simulink model "ImpedanceControl"  (R2017a)
settings: Solver=VariableStepAuto  StartTime=0.0  StopTime=10.0  RelTol=1e-3
libraries: mblibv1 x60
(part 2 of 2)

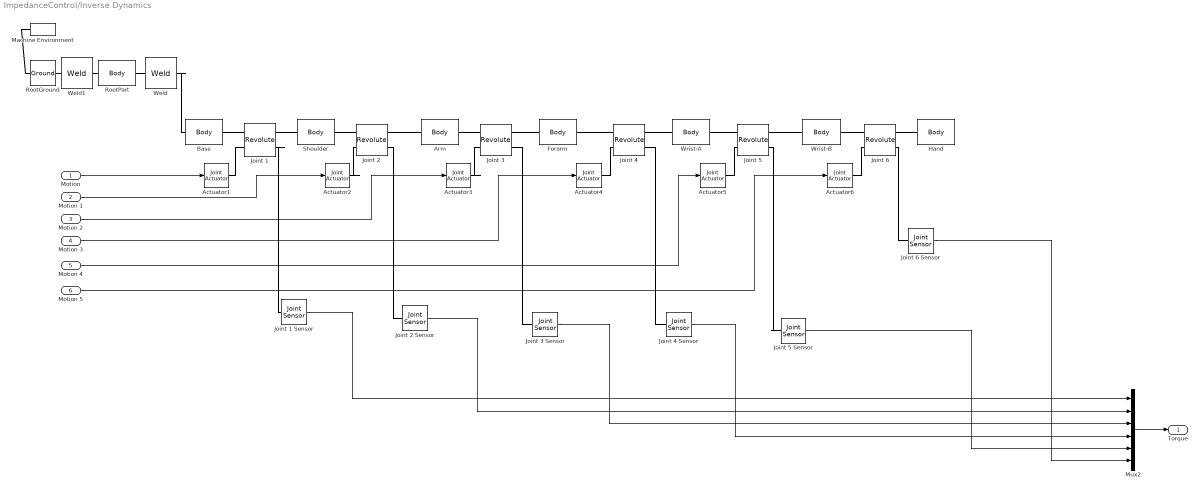
== system ImpedanceControl/Inverse Dynamics  ==
  "Motion " : Inport
  Motion 1 : Inport  Port=2
  Motion 2 : Inport  Port=3
  Motion 3 : Inport  Port=4
  Motion 4 : Inport  Port=5
  Motion 5 : Inport  Port=6
  Actuator{1..6} (6 alike) : mblibv1/Sensors &  Actuators/Joint Actuator  UpdateFromCAD=off  PhysicalDomain=Mechanical  PortType=blob  ActuationStyle=Motion  AngleUnits=deg  ArcVelocityUnits=deg/s  ArcAccelerationUnits=deg/s^2  CoordPositionUnits=m  VelocityUnits=m/s  AccelerationUnits=m/s^2  ForceUnits=N  TorqueUnits=N*m  ActiveIO=on  Width=3  DialogClass=MechanicalActuatorBlock  Primitive=R1  ReferenceFrame=Absolute (World)
      settings: SourceProductName=Simscape Multibody  SourceProductBaseCode=MS
  Arm : mblibv1/Bodies/Body  LConnTagsString=CS2  RConnTagsString=CS3  UpdateFromCAD=on  DialogClass=MechanicalBodyBlock  Mass=1.056  MassUnits=kg  InertiaUnits=kg*m^2  Inertia=[0.0375645,-1.33324e-07,0.000108785;-1.33324e-07,0.0372402,-2.39225e-07;0.000108785,-2.39225e-07,0.00059301]  Shape=Cylinder  ShapeDims=[1 1]  ShapeUnits=m  ShapeUse=false  Density=1  DensityUnits=kg/m^3  DensityUse=false  GraphicsMode=GFXFILE  GraphicsFileName=Jaco_3_7 - arm_ass-1.STL  BodyColorSelMode=COLORPALETTE  BodyColor=[0.752941;0.752941;0.752941]  AttachedToCS=CS1  CG=Right$CG$[0.10282 0.0944444 0.508793]$WORLD$WORLD$m$[0.695251 0.715707 -0.0662524;0.718767 -0.692291 0.0640847;0 -0.092175 -0.995743]$3x3 Transform$rad$WORLD$false$none  WorkingFrames=Right$CS1$[-0.183907 0.105598 0.903425]$WORLD$WORLD$m$[0.695251 0.715707 -0.0662524;0.718767 -0.692291 0.0640847;0 -0.092175 -0.995743]$3x3 Transform$rad$WORLD$false$none#Left$CS2$[0.0767642 0.095252 0.300589]$WORLD$WORLD$m$[1 0 0;0 1 0;0 0 1]$3x3 Transform$rad$WORLD$true$none#Right$CS3$[0.10358 0.0686179 0.708843]$WORLD$WORLD$m$[1 0 0;0 1 0;0 0 1]$3x3 Transform$rad$WORLD$true$none  CGPos=[0.10282 0.0944444 0.508793]  CGRot=[0.695251 0.715707 -0.0662524;0.718767 -0.692291 0.0640847;0 -0.092175 -0.995743]  CS0Pos=[]  CS0Rot=[]  CS1Pos=[-0.183907 0.105598 0.903425]  CS1Rot=[0.695251 0.715707 -0.0662524;0.718767 -0.692291 0.0640847;0 -0.092175 -0.995743]  CS2Pos=[0.0767642 0.095252 0.300589]  CS2Rot=[1 0 0;0 1 0;0 0 1]  CS3Pos=[0.10358 0.0686179 0.708843]  CS3Rot=[1 0 0;0 1 0;0 0 1]  CS4Pos=[]  CS4Rot=[]  CS5Pos=[]  CS5Rot=[]  CS6Pos=[]  CS6Rot=[]  CS7Pos=[]  CS7Rot=[]  CS8Pos=[]  CS8Rot=[]  CS9Pos=[]  CS9Rot=[]  CS10Pos=[]  CS10Rot=[]  CS11Pos=[]  CS11Rot=[]  CS12Pos=[]  CS12Rot=[]  CS13Pos=[]  CS13Rot=[]  CS14Pos=[]  CS14Rot=[]  CS15Pos=[]  CS15Rot=[]  CS16Pos=[]  CS16Rot=[]  CS17Pos=[]  CS17Rot=[]  CS18Pos=[]  CS18Rot=[]  CS19Pos=[]  CS19Rot=[]  CS20Pos=[]  CS20Rot=[]
      settings: SourceProductName=Simscape Multibody  SourceProductBaseCode=MS
  Base : mblibv1/Bodies/Body  LConnTagsString=CS2  RConnTagsString=CS3  UpdateFromCAD=on  DialogClass=MechanicalBodyBlock  Mass=0.570939  MassUnits=kg  InertiaUnits=kg*m^2  Inertia=[0.00175947,1.92772e-07,-3.1782e-05;1.92772e-07,0.00176256,-3.18122e-05;-3.1782e-05,-3.18122e-05,0.000478232]  Shape=Cylinder  ShapeDims=[1 1]  ShapeUnits=m  ShapeUse=false  Density=1  DensityUnits=kg/m^3  DensityUse=false  GraphicsMode=GFXFILE  GraphicsFileName=Jaco_3_7 - base_ass-1.STL  BodyColorSelMode=COLORPALETTE  BodyColor=[0.752941;0.752941;0.752941]  AttachedToCS=CS1  CG=Right$CG$[0.0747134 0.093124 0.128067]$WORLD$WORLD$m$[1 0 0;0 1 0;0 0 1]$3x3 Transform$rad$WORLD$false$none  WorkingFrames=Right$CS1$[0.106448 0.0299726 -0.0762042]$WORLD$WORLD$m$[1 0 0;0 1 0;0 0 1]$3x3 Transform$rad$WORLD$false$none#Left$CS2$[0.0747134 0.093124 0.128067]$WORLD$WORLD$m$[1 0 0;0 1 0;0 0 1]$3x3 Transform$rad$WORLD$true$none#Right$CS3$[0.0753736 0.0938145 0.182089]$WORLD$WORLD$m$[1 0 0;0 1 0;0 0 1]$3x3 Transform$rad$WORLD$true$none  CGPos=[0.0747134 0.093124 0.128067]  CGRot=[1 0 0;0 1 0;0 0 1]  CS0Pos=[]  CS0Rot=[]  CS1Pos=[0.106448 0.0299726 -0.0762042]  CS1Rot=[1 0 0;0 1 0;0 0 1]  CS2Pos=[0.0747134 0.093124 0.128067]  CS2Rot=[1 0 0;0 1 0;0 0 1]  CS3Pos=[0.0753736 0.0938145 0.182089]  CS3Rot=[1 0 0;0 1 0;0 0 1]  CS4Pos=[]  CS4Rot=[]  CS5Pos=[]  CS5Rot=[]  CS6Pos=[]  CS6Rot=[]  CS7Pos=[]  CS7Rot=[]  CS8Pos=[]  CS8Rot=[]  CS9Pos=[]  CS9Rot=[]  CS10Pos=[]  CS10Rot=[]  CS11Pos=[]  CS11Rot=[]  CS12Pos=[]  CS12Rot=[]  CS13Pos=[]  CS13Rot=[]  CS14Pos=[]  CS14Rot=[]  CS15Pos=[]  CS15Rot=[]  CS16Pos=[]  CS16Rot=[]  CS17Pos=[]  CS17Rot=[]  CS18Pos=[]  CS18Rot=[]  CS19Pos=[]  CS19Rot=[]  CS20Pos=[]  CS20Rot=[]
      settings: SourceProductName=Simscape Multibody  SourceProductBaseCode=MS
  Forarm : mblibv1/Bodies/Body  LConnTagsString=CS2  RConnTagsString=CS3  UpdateFromCAD=on  DialogClass=MechanicalBodyBlock  Mass=0.735414  MassUnits=kg  InertiaUnits=kg*m^2  Inertia=[0.00626271,-0.000115651,1.81814e-08;-0.000115651,0.000377159,4.13244e-07;1.81814e-08,4.13244e-07,0.00610747]  Shape=Cylinder  ShapeDims=[1 1]  ShapeUnits=m  ShapeUse=false  Density=1  DensityUnits=kg/m^3  DensityUse=false  GraphicsMode=GFXFILE  GraphicsFileName=Jaco_3_7 - forarm_ass-1.STL  BodyColorSelMode=COLORPALETTE  BodyColor=[0.752941;0.752941;0.752941]  AttachedToCS=CS1  CG=Right$CG$[0.142291 0.0111153 0.740623]$WORLD$WORLD$m$[0.695251 0.650811 0.305076;0.718767 -0.629518 -0.295094;0 0.424443 -0.905455]$3x3 Transform$rad$WORLD$false$none  WorkingFrames=Right$CS1$[-0.0310579 0.0970807 0.899014]$WORLD$WORLD$m$[0.695251 0.650811 0.305076;0.718767 -0.629518 -0.295094;0 0.424443 -0.905455]$3x3 Transform$rad$WORLD$false$none#Left$CS2$[0.10358 0.0686179 0.708843]$WORLD$WORLD$m$[1 0 0;0 1 0;0 0 1]$3x3 Transform$rad$WORLD$true$none#Right$CS3$[0.230802 -0.0700932 0.796915]$WORLD$WORLD$m$[1 0 0;0 1 0;0 0 1]$3x3 Transform$rad$WORLD$true$none  CGPos=[0.142291 0.0111153 0.740623]  CGRot=[0.695251 0.650811 0.305076;0.718767 -0.629518 -0.295094;0 0.424443 -0.905455]  CS0Pos=[]  CS0Rot=[]  CS1Pos=[-0.0310579 0.0970807 0.899014]  CS1Rot=[0.695251 0.650811 0.305076;0.718767 -0.629518 -0.295094;0 0.424443 -0.905455]  CS2Pos=[0.10358 0.0686179 0.708843]  CS2Rot=[1 0 0;0 1 0;0 0 1]  CS3Pos=[0.230802 -0.0700932 0.796915]  CS3Rot=[1 0 0;0 1 0;0 0 1]  CS4Pos=[]  CS4Rot=[]  CS5Pos=[]  CS5Rot=[]  CS6Pos=[]  CS6Rot=[]  CS7Pos=[]  CS7Rot=[]  CS8Pos=[]  CS8Rot=[]  CS9Pos=[]  CS9Rot=[]  CS10Pos=[]  CS10Rot=[]  CS11Pos=[]  CS11Rot=[]  CS12Pos=[]  CS12Rot=[]  CS13Pos=[]  CS13Rot=[]  CS14Pos=[]  CS14Rot=[]  CS15Pos=[]  CS15Rot=[]  CS16Pos=[]  CS16Rot=[]  CS17Pos=[]  CS17Rot=[]  CS18Pos=[]  CS18Rot=[]  CS19Pos=[]  CS19Rot=[]  CS20Pos=[]  CS20Rot=[]
      settings: SourceProductName=Simscape Multibody  SourceProductBaseCode=MS
  Hand : mblibv1/Bodies/Body  LConnTagsString=CS2  UpdateFromCAD=on  DialogClass=MechanicalBodyBlock  Mass=0.395999  MassUnits=kg  InertiaUnits=kg*m^2  Inertia=[0.00124769,-0.000197969,-5.51354e-06;-0.000197969,0.000409818,-2.12169e-05;-5.51354e-06,-2.12169e-05,0.00139509]  Shape=Cylinder  ShapeDims=[1 1]  ShapeUnits=m  ShapeUse=false  Density=1  DensityUnits=kg/m^3  DensityUse=false  GraphicsMode=GFXFILE  GraphicsFileName=Jaco_3_7 - Hand_ass-1.STL  BodyColorSelMode=COLORPALETTE  BodyColor=[0.752941;0.752941;0.752941]  AttachedToCS=CS1  CG=Right$CG$[0.35442 -0.232757 0.799495]$WORLD$WORLD$m$[-0.439555 0.858973 -0.262597;-0.828489 -0.500657 -0.250895;-0.346983 0.107276 0.931716]$3x3 Transform$rad$WORLD$false$none  WorkingFrames=Right$CS1$[0.362295 -0.115327 0.65151]$WORLD$WORLD$m$[-0.439555 0.858973 -0.262597;-0.828489 -0.500657 -0.250895;-0.346983 0.107276 0.931716]$3x3 Transform$rad$WORLD$false$none#Left$CS2$[0.306767 -0.196631 0.795235]$WORLD$WORLD$m$[1 0 0;0 1 0;0 0 1]$3x3 Transform$rad$WORLD$true$none  CGPos=[0.35442 -0.232757 0.799495]  CGRot=[-0.439555 0.858973 -0.262597;-0.828489 -0.500657 -0.250895;-0.346983 0.107276 0.931716]  CS0Pos=[]  CS0Rot=[]  CS1Pos=[0.362295 -0.115327 0.65151]  CS1Rot=[-0.439555 0.858973 -0.262597;-0.828489 -0.500657 -0.250895;-0.346983 0.107276 0.931716]  CS2Pos=[0.306767 -0.196631 0.795235]  CS2Rot=[1 0 0;0 1 0;0 0 1]  CS3Pos=[]  CS3Rot=[]  CS4Pos=[]  CS4Rot=[]  CS5Pos=[]  CS5Rot=[]  CS6Pos=[]  CS6Rot=[]  CS7Pos=[]  CS7Rot=[]  CS8Pos=[]  CS8Rot=[]  CS9Pos=[]  CS9Rot=[]  CS10Pos=[]  CS10Rot=[]  CS11Pos=[]  CS11Rot=[]  CS12Pos=[]  CS12Rot=[]  CS13Pos=[]  CS13Rot=[]  CS14Pos=[]  CS14Rot=[]  CS15Pos=[]  CS15Rot=[]  CS16Pos=[]  CS16Rot=[]  CS17Pos=[]  CS17Rot=[]  CS18Pos=[]  CS18Rot=[]  CS19Pos=[]  CS19Rot=[]  CS20Pos=[]  CS20Rot=[]
      settings: SourceProductName=Simscape Multibody  SourceProductBaseCode=MS
  Joint 1 : mblibv1/Joints/Revolute  LConnTagsString=__newl0|SA1  RConnTagsString=__newr0|SA1  UpdateFromCAD=on  NumSAPorts=2  CutJoint=off  MarkAsCut=off  Primitives=prismatic  PrimitiveProps=R1$World$[0,0,1]$revolute  DialogClass=JointBlock  R1Axis=[0,0,1]
      settings: SourceProductName=Simscape Multibody  SourceProductBaseCode=MS
  Joint 1 Sensor : mblibv1/Sensors &  Actuators/Joint Sensor  UpdateFromCAD=off  PhysicalDomain=Mechanical  PortType=blob  Muxed=off  Pose=off  Angle=off  AngleUnits=deg  ArcVelocity=off  ArcVelocityUnits=deg/s  ArcAcceleration=off  ArcAccelerationUnits=deg/s^2  CoordPosition=on  CoordPositionUnits=m  Velocity=off  VelocityUnits=m/s  Acceleration=off  AccelerationUnits=m/s^2  Quaternion=on  QuaternionDT=off  QuaternionDDT=off  QuaternionUnits=off  OutputVector=[1]  ActiveIO=on  Width=1  DialogClass=MechanicalSensorBlock  Primitive=R1  Force=off  ForceUnits=N  Torque=on  TorqueUnits=N*m  ReferenceFrame=Absolute (World)  ReactionSensedSide=Base  ReactionReferenceFrame=Absolute (World)  ReactionForce=off  ReactionForceUnits=N  ReactionMoment=off  ReactionMomentUnits=N*m
      settings: SourceProductName=Simscape Multibody  SourceProductBaseCode=MS
  Joint 2 : mblibv1/Joints/Revolute  LConnTagsString=__newl0|SA1  RConnTagsString=__newr0|SA1  UpdateFromCAD=on  NumSAPorts=2  CutJoint=off  MarkAsCut=off  Primitives=prismatic  PrimitiveProps=R1$World$[0.695251,0.718767,0]$revolute  DialogClass=JointBlock  R1Axis=[0.695251,0.718767,0]
      settings: SourceProductName=Simscape Multibody  SourceProductBaseCode=MS
  Joint 2 Sensor : mblibv1/Sensors &  Actuators/Joint Sensor  UpdateFromCAD=off  PhysicalDomain=Mechanical  PortType=blob  Muxed=off  Pose=off  Angle=off  AngleUnits=deg  ArcVelocity=off  ArcVelocityUnits=deg/s  ArcAcceleration=off  ArcAccelerationUnits=deg/s^2  CoordPosition=on  CoordPositionUnits=m  Velocity=off  VelocityUnits=m/s  Acceleration=off  AccelerationUnits=m/s^2  Quaternion=on  QuaternionDT=off  QuaternionDDT=off  QuaternionUnits=off  OutputVector=[1]  ActiveIO=on  Width=1  DialogClass=MechanicalSensorBlock  Primitive=R1  Force=off  ForceUnits=N  Torque=on  TorqueUnits=N*m  ReferenceFrame=Absolute (World)  ReactionSensedSide=Base  ReactionReferenceFrame=Absolute (World)  ReactionForce=off  ReactionForceUnits=N  ReactionMoment=off  ReactionMomentUnits=N*m
      settings: SourceProductName=Simscape Multibody  SourceProductBaseCode=MS
  Joint 3 : mblibv1/Joints/Revolute  LConnTagsString=__newl0|SA1  RConnTagsString=__newr0|SA1  UpdateFromCAD=on  NumSAPorts=2  CutJoint=off  MarkAsCut=off  Primitives=prismatic  PrimitiveProps=R1$World$[-0.695251,-0.718767,0]$revolute  DialogClass=JointBlock  R1Axis=[-0.695251,-0.718767,0]
      settings: SourceProductName=Simscape Multibody  SourceProductBaseCode=MS
  Joint 3 Sensor : mblibv1/Sensors &  Actuators/Joint Sensor  UpdateFromCAD=off  PhysicalDomain=Mechanical  PortType=blob  Muxed=off  Pose=off  Angle=off  AngleUnits=deg  ArcVelocity=off  ArcVelocityUnits=deg/s  ArcAcceleration=off  ArcAccelerationUnits=deg/s^2  CoordPosition=on  CoordPositionUnits=m  Velocity=off  VelocityUnits=m/s  Acceleration=off  AccelerationUnits=m/s^2  Quaternion=on  QuaternionDT=off  QuaternionDDT=off  QuaternionUnits=off  OutputVector=[1]  ActiveIO=on  Width=1  DialogClass=MechanicalSensorBlock  Primitive=R1  Force=off  ForceUnits=N  Torque=on  TorqueUnits=N*m  ReferenceFrame=Absolute (World)  ReactionSensedSide=Base  ReactionReferenceFrame=Absolute (World)  ReactionForce=off  ReactionForceUnits=N  ReactionMoment=off  ReactionMomentUnits=N*m
      settings: SourceProductName=Simscape Multibody  SourceProductBaseCode=MS
  Joint 4 : mblibv1/Joints/Revolute  LConnTagsString=__newl0|SA1  RConnTagsString=__newr0|SA1  UpdateFromCAD=on  NumSAPorts=2  CutJoint=off  MarkAsCut=off  Primitives=prismatic  PrimitiveProps=R1$World$[0.650811,-0.629518,0.424443]$revolute  DialogClass=JointBlock  R1Axis=[0.650811,-0.629518,0.424443]
      settings: SourceProductName=Simscape Multibody  SourceProductBaseCode=MS
  Joint 4 Sensor : mblibv1/Sensors &  Actuators/Joint Sensor  UpdateFromCAD=off  PhysicalDomain=Mechanical  PortType=blob  Muxed=off  Pose=off  Angle=off  AngleUnits=deg  ArcVelocity=off  ArcVelocityUnits=deg/s  ArcAcceleration=off  ArcAccelerationUnits=deg/s^2  CoordPosition=on  CoordPositionUnits=m  Velocity=off  VelocityUnits=m/s  Acceleration=off  AccelerationUnits=m/s^2  Quaternion=on  QuaternionDT=off  QuaternionDDT=off  QuaternionUnits=off  OutputVector=[1]  ActiveIO=on  Width=1  DialogClass=MechanicalSensorBlock  Primitive=R1  Force=off  ForceUnits=N  Torque=on  TorqueUnits=N*m  ReferenceFrame=Absolute (World)  ReactionSensedSide=Base  ReactionReferenceFrame=Absolute (World)  ReactionForce=off  ReactionForceUnits=N  ReactionMoment=off  ReactionMomentUnits=N*m
      settings: SourceProductName=Simscape Multibody  SourceProductBaseCode=MS
  Joint 5 : mblibv1/Joints/Revolute  LConnTagsString=__newl0|SA1  RConnTagsString=__newr0|SA1  UpdateFromCAD=on  NumSAPorts=2  CutJoint=off  MarkAsCut=off  Primitives=prismatic  PrimitiveProps=R1$World$[0.15169,-0.946456,-0.284976]$revolute  DialogClass=JointBlock  R1Axis=[0.15169,-0.946456,-0.284976]
      settings: SourceProductName=Simscape Multibody  SourceProductBaseCode=MS
  Joint 5 Sensor : mblibv1/Sensors &  Actuators/Joint Sensor  UpdateFromCAD=off  PhysicalDomain=Mechanical  PortType=blob  Muxed=off  Pose=off  Angle=off  AngleUnits=deg  ArcVelocity=off  ArcVelocityUnits=deg/s  ArcAcceleration=off  ArcAccelerationUnits=deg/s^2  CoordPosition=on  CoordPositionUnits=m  Velocity=off  VelocityUnits=m/s  Acceleration=off  AccelerationUnits=m/s^2  Quaternion=on  QuaternionDT=off  QuaternionDDT=off  QuaternionUnits=off  OutputVector=[1]  ActiveIO=on  Width=1  DialogClass=MechanicalSensorBlock  Primitive=R1  Force=off  ForceUnits=N  Torque=on  TorqueUnits=N*m  ReferenceFrame=Absolute (World)  ReactionSensedSide=Base  ReactionReferenceFrame=Absolute (World)  ReactionForce=off  ReactionForceUnits=N  ReactionMoment=off  ReactionMomentUnits=N*m
      settings: SourceProductName=Simscape Multibody  SourceProductBaseCode=MS
  Joint 6 : mblibv1/Joints/Revolute  LConnTagsString=__newl0|SA1  RConnTagsString=__newr0|SA1  UpdateFromCAD=on  NumSAPorts=2  CutJoint=off  MarkAsCut=off  Primitives=prismatic  PrimitiveProps=R1$World$[0.858973,-0.500657,0.107276]$revolute  DialogClass=JointBlock  R1Axis=[0.858973,-0.500657,0.107276]
      settings: SourceProductName=Simscape Multibody  SourceProductBaseCode=MS
  Joint 6 Sensor : mblibv1/Sensors &  Actuators/Joint Sensor  UpdateFromCAD=off  PhysicalDomain=Mechanical  PortType=blob  Muxed=off  Pose=off  Angle=off  AngleUnits=deg  ArcVelocity=off  ArcVelocityUnits=deg/s  ArcAcceleration=off  ArcAccelerationUnits=deg/s^2  CoordPosition=on  CoordPositionUnits=m  Velocity=off  VelocityUnits=m/s  Acceleration=off  AccelerationUnits=m/s^2  Quaternion=on  QuaternionDT=off  QuaternionDDT=off  QuaternionUnits=off  OutputVector=[1]  ActiveIO=on  Width=1  DialogClass=MechanicalSensorBlock  Primitive=R1  Force=off  ForceUnits=N  Torque=on  TorqueUnits=N*m  ReferenceFrame=Absolute (World)  ReactionSensedSide=Base  ReactionReferenceFrame=Absolute (World)  ReactionForce=off  ReactionForceUnits=N  ReactionMoment=off  ReactionMomentUnits=N*m
      settings: SourceProductName=Simscape Multibody  SourceProductBaseCode=MS
  Machine Environment : mblibv1/Bodies/Machine Environment  PortType=env  PhysicalDomain=Mechanical  DialogTemplateClass=MECH.MachineEnvironment  SyncWhenCopied=off  Gravity=[0 0 -9.81]  GravityUnits=m/s^2  GravityAsSignal=off  Dimensionality=Auto-detect  AnalysisType=Inverse dynamics  LinearAssemblyTolerance=1e-3  LinearAssemblyToleranceUnits=m  AngularAssemblyTolerance=1e-3  AngularAssemblyToleranceUnits=rad  ConstraintSolverType=Stabilizing  ConstraintRelTolerance=1e-4  ConstraintAbsTolerance=1e-4  UseRobustSingularityHandling=off  RedundancyAnalysisToleranceType=Automatically select tolerance  RedundancyAnalysisTolerance=1e-14  StatePerturbationType=Fixed  PerturbationSize=1e-5  VisualizeMachine=on  BodyVisualizationType=Use model default body geometries  BodyColorSelMode=Use model default  DefaultBodyColor=[1 0 0]
      settings: SourceProductName=Simscape Multibody  SourceProductBaseCode=MS
  Mux2 : Mux  Inputs=6
  RootGround : mblibv1/Bodies/Ground  UpdateFromCAD=on  LeftPortType=env  RightPortType=workingframe  PhysicalDomain=Mechanical  DialogClass=GroundBlock  CoordPosition=[0.154743,0.00421299,0.535333]  CoordPositionUnits=m  StateVectorMgrId=-1  MachineId=[0 0]  ShowEnvPort=on  ParameterChecksum=[2113353881, 666478824, 1095862328, 2132002380]  TopologyChecksum=[2383253151, 3882554260, 534595173, 222725373]
      settings: SourceProductName=Simscape Multibody  SourceProductBaseCode=MS
  RootPart : mblibv1/Bodies/Body  LConnTagsString=CS3  RConnTagsString=CS2  UpdateFromCAD=on  DialogClass=MechanicalBodyBlock  Mass=0  MassUnits=kg  InertiaUnits=kg*m^2  Inertia=[0,0,0;0,0,0;0,0,0]  Shape=Cylinder  ShapeDims=[1 1]  ShapeUnits=m  ShapeUse=false  Density=1  DensityUnits=kg/m^3  DensityUse=false  GraphicsMode=MACHINE_DEFAULT  BodyColorSelMode=MACHINE_DEFAULT  BodyColor=[1;0;0]  AttachedToCS=CS1  CG=Right$CG$[0.154743 0.00421299 0.535333]$WORLD$WORLD$m$[1 0 0;0 1 0;0 0 1]$3x3 Transform$rad$WORLD$false$none  WorkingFrames=Right$CS1$[0 0 0]$WORLD$WORLD$m$[1 0 0;0 1 0;0 0 1]$3x3 Transform$rad$WORLD$false$none#Right$CS2$[0.0747134 0.093124 0.128067]$WORLD$WORLD$m$[1 0 0;0 1 0;0 0 1]$3x3 Transform$rad$WORLD$true$none#Left$CS3$[0.154743 0.00421299 0.535333]$WORLD$WORLD$m$[1 0 0;0 1 0;0 0 1]$3x3 Transform$rad$WORLD$true$none  CGPos=[0.154743 0.00421299 0.535333]  CGRot=[1 0 0;0 1 0;0 0 1]  CS0Pos=[]  CS0Rot=[]  CS1Pos=[0 0 0]  CS1Rot=[1 0 0;0 1 0;0 0 1]  CS2Pos=[0.0747134 0.093124 0.128067]  CS2Rot=[1 0 0;0 1 0;0 0 1]  CS3Pos=[0.154743 0.00421299 0.535333]  CS3Rot=[1 0 0;0 1 0;0 0 1]  CS4Pos=[]  CS4Rot=[]  CS5Pos=[]  CS5Rot=[]  CS6Pos=[]  CS6Rot=[]  CS7Pos=[]  CS7Rot=[]  CS8Pos=[]  CS8Rot=[]  CS9Pos=[]  CS9Rot=[]  CS10Pos=[]  CS10Rot=[]  CS11Pos=[]  CS11Rot=[]  CS12Pos=[]  CS12Rot=[]  CS13Pos=[]  CS13Rot=[]  CS14Pos=[]  CS14Rot=[]  CS15Pos=[]  CS15Rot=[]  CS16Pos=[]  CS16Rot=[]  CS17Pos=[]  CS17Rot=[]  CS18Pos=[]  CS18Rot=[]  CS19Pos=[]  CS19Rot=[]  CS20Pos=[]  CS20Rot=[]
      settings: SourceProductName=Simscape Multibody  SourceProductBaseCode=MS
  Shoulder : mblibv1/Bodies/Body  LConnTagsString=CS3  RConnTagsString=CS2  UpdateFromCAD=on  DialogClass=MechanicalBodyBlock  Mass=0.813994  MassUnits=kg  InertiaUnits=kg*m^2  Inertia=[0.0026546,0.000304923,5.38935e-08;0.000304923,0.000595598,-3.17242e-07;5.38935e-08,-3.17242e-07,0.00258406]  Shape=Cylinder  ShapeDims=[1 1]  ShapeUnits=m  ShapeUse=false  Density=1  DensityUnits=kg/m^3  DensityUse=false  GraphicsMode=GFXFILE  GraphicsFileName=Jaco_3_7 - shoulder_ass-1.STL  BodyColorSelMode=COLORPALETTE  BodyColor=[0.752941;0.752941;0.752941]  AttachedToCS=CS1  CG=Right$CG$[0.0698164 0.0880634 0.250193]$WORLD$WORLD$m$[0.695251 0 0.718767;0.718767 0 -0.695251;0 1 0]$3x3 Transform$rad$WORLD$false$none  WorkingFrames=Right$CS1$[-0.0564522 0.142463 0.184725]$WORLD$WORLD$m$[0.695251 0 0.718767;0.718767 0 -0.695251;0 1 0]$3x3 Transform$rad$WORLD$false$none#Right$CS2$[0.0767642 0.095252 0.300589]$WORLD$WORLD$m$[1 0 0;0 1 0;0 0 1]$3x3 Transform$rad$WORLD$true$none#Left$CS3$[0.0753736 0.0938145 0.182089]$WORLD$WORLD$m$[1 0 0;0 1 0;0 0 1]$3x3 Transform$rad$WORLD$true$none  CGPos=[0.0698164 0.0880634 0.250193]  CGRot=[0.695251 0 0.718767;0.718767 0 -0.695251;0 1 0]  CS0Pos=[]  CS0Rot=[]  CS1Pos=[-0.0564522 0.142463 0.184725]  CS1Rot=[0.695251 0 0.718767;0.718767 0 -0.695251;0 1 0]  CS2Pos=[0.0767642 0.095252 0.300589]  CS2Rot=[1 0 0;0 1 0;0 0 1]  CS3Pos=[0.0753736 0.0938145 0.182089]  CS3Rot=[1 0 0;0 1 0;0 0 1]  CS4Pos=[]  CS4Rot=[]  CS5Pos=[]  CS5Rot=[]  CS6Pos=[]  CS6Rot=[]  CS7Pos=[]  CS7Rot=[]  CS8Pos=[]  CS8Rot=[]  CS9Pos=[]  CS9Rot=[]  CS10Pos=[]  CS10Rot=[]  CS11Pos=[]  CS11Rot=[]  CS12Pos=[]  CS12Rot=[]  CS13Pos=[]  CS13Rot=[]  CS14Pos=[]  CS14Rot=[]  CS15Pos=[]  CS15Rot=[]  CS16Pos=[]  CS16Rot=[]  CS17Pos=[]  CS17Rot=[]  CS18Pos=[]  CS18Rot=[]  CS19Pos=[]  CS19Rot=[]  CS20Pos=[]  CS20Rot=[]
      settings: SourceProductName=Simscape Multibody  SourceProductBaseCode=MS
  Weld : mblibv1/Joints/Weld  LConnTagsString=__newl0  RConnTagsString=__newr0  UpdateFromCAD=on  NumSAPorts=0  CutJoint=off  MarkAsCut=off  Primitives=weld  PrimitiveProps=W$WORLD$[0.57735,0.57735,0.57735]$weld  DialogClass=JointBlock  WAxis=[0.57735,0.57735,0.57735]
      settings: SourceProductName=Simscape Multibody  SourceProductBaseCode=MS
  Weld1 : mblibv1/Joints/Weld  LConnTagsString=__newl0  RConnTagsString=__newr0  UpdateFromCAD=on  NumSAPorts=0  CutJoint=off  MarkAsCut=off  Primitives=weld  PrimitiveProps=W$WORLD$[0.57735,0.57735,0.57735]$weld  DialogClass=JointBlock  WAxis=[0.57735,0.57735,0.57735]
      settings: SourceProductName=Simscape Multibody  SourceProductBaseCode=MS
  Wrist-A : mblibv1/Bodies/Body  LConnTagsString=CS3  RConnTagsString=CS2  UpdateFromCAD=on  DialogClass=MechanicalBodyBlock  Mass=0.44698  MassUnits=kg  InertiaUnits=kg*m^2  Inertia=[0.000407036,-3.06246e-08,5.0605e-09;-3.06246e-08,0.000239744,-8.7175e-05;5.0605e-09,-8.7175e-05,0.000376656]  Shape=Cylinder  ShapeDims=[1 1]  ShapeUnits=m  ShapeUse=false  Density=1  DensityUnits=kg/m^3  DensityUse=false  GraphicsMode=GFXFILE  GraphicsFileName=Jaco_3_7 - wrist1_ass-1.STL  BodyColorSelMode=COLORPALETTE  BodyColor=[0.752941;0.752941;0.752941]  AttachedToCS=CS1  CG=Right$CG$[0.251866 -0.101707 0.805258]$WORLD$WORLD$m$[0.709409 0.650811 -0.270524;0.30501 -0.629518 -0.714616;-0.63538 0.424443 -0.64509]$3x3 Transform$rad$WORLD$false$none  WorkingFrames=Right$CS1$[0.228148 -0.0304193 0.852839]$WORLD$WORLD$m$[0.709409 0.650811 -0.270524;0.30501 -0.629518 -0.714616;-0.63538 0.424443 -0.64509]$3x3 Transform$rad$WORLD$false$none#Right$CS2$[0.264276 -0.136155 0.802577]$WORLD$WORLD$m$[1 0 0;0 1 0;0 0 1]$3x3 Transform$rad$WORLD$true$none#Left$CS3$[0.230802 -0.0700932 0.796915]$WORLD$WORLD$m$[1 0 0;0 1 0;0 0 1]$3x3 Transform$rad$WORLD$true$none  CGPos=[0.251866 -0.101707 0.805258]  CGRot=[0.709409 0.650811 -0.270524;0.30501 -0.629518 -0.714616;-0.63538 0.424443 -0.64509]  CS0Pos=[]  CS0Rot=[]  CS1Pos=[0.228148 -0.0304193 0.852839]  CS1Rot=[0.709409 0.650811 -0.270524;0.30501 -0.629518 -0.714616;-0.63538 0.424443 -0.64509]  CS2Pos=[0.264276 -0.136155 0.802577]  CS2Rot=[1 0 0;0 1 0;0 0 1]  CS3Pos=[0.230802 -0.0700932 0.796915]  CS3Rot=[1 0 0;0 1 0;0 0 1]  CS4Pos=[]  CS4Rot=[]  CS5Pos=[]  CS5Rot=[]  CS6Pos=[]  CS6Rot=[]  CS7Pos=[]  CS7Rot=[]  CS8Pos=[]  CS8Rot=[]  CS9Pos=[]  CS9Rot=[]  CS10Pos=[]  CS10Rot=[]  CS11Pos=[]  CS11Rot=[]  CS12Pos=[]  CS12Rot=[]  CS13Pos=[]  CS13Rot=[]  CS14Pos=[]  CS14Rot=[]  CS15Pos=[]  CS15Rot=[]  CS16Pos=[]  CS16Rot=[]  CS17Pos=[]  CS17Rot=[]  CS18Pos=[]  CS18Rot=[]  CS19Pos=[]  CS19Rot=[]  CS20Pos=[]  CS20Rot=[]
      settings: SourceProductName=Simscape Multibody  SourceProductBaseCode=MS
  Wrist-B : mblibv1/Bodies/Body  LConnTagsString=CS3  RConnTagsString=CS2  UpdateFromCAD=on  DialogClass=MechanicalBodyBlock  Mass=0.44698  MassUnits=kg  InertiaUnits=kg*m^2  Inertia=[0.000407036,-3.06246e-08,5.0605e-09;-3.06246e-08,0.000239744,-8.7175e-05;5.0605e-09,-8.7175e-05,0.000376656]  Shape=Cylinder  ShapeDims=[1 1]  ShapeUnits=m  ShapeUse=false  Density=1  DensityUnits=kg/m^3  DensityUse=false  GraphicsMode=GFXFILE  GraphicsFileName=Jaco_3_7 - wrist2_ass-1.STL  BodyColorSelMode=COLORPALETTE  BodyColor=[0.752941;0.752941;0.752941]  AttachedToCS=CS1  CG=Right$CG$[0.28076 -0.170724 0.795794]$WORLD$WORLD$m$[-0.298122 0.15169 0.942398;-0.318695 -0.946456 0.0515257;0.899754 -0.284976 0.330502]$3x3 Transform$rad$WORLD$false$none  WorkingFrames=Right$CS1$[0.211333 -0.128563 0.759589]$WORLD$WORLD$m$[-0.298122 0.15169 0.942398;-0.318695 -0.946456 0.0515257;0.899754 -0.284976 0.330502]$3x3 Transform$rad$WORLD$false$none#Right$CS2$[0.306767 -0.196631 0.795235]$WORLD$WORLD$m$[1 0 0;0 1 0;0 0 1]$3x3 Transform$rad$WORLD$true$none#Left$CS3$[0.264276 -0.136155 0.802577]$WORLD$WORLD$m$[1 0 0;0 1 0;0 0 1]$3x3 Transform$rad$WORLD$true$none  CGPos=[0.28076 -0.170724 0.795794]  CGRot=[-0.298122 0.15169 0.942398;-0.318695 -0.946456 0.0515257;0.899754 -0.284976 0.330502]  CS0Pos=[]  CS0Rot=[]  CS1Pos=[0.211333 -0.128563 0.759589]  CS1Rot=[-0.298122 0.15169 0.942398;-0.318695 -0.946456 0.0515257;0.899754 -0.284976 0.330502]  CS2Pos=[0.306767 -0.196631 0.795235]  CS2Rot=[1 0 0;0 1 0;0 0 1]  CS3Pos=[0.264276 -0.136155 0.802577]  CS3Rot=[1 0 0;0 1 0;0 0 1]  CS4Pos=[]  CS4Rot=[]  CS5Pos=[]  CS5Rot=[]  CS6Pos=[]  CS6Rot=[]  CS7Pos=[]  CS7Rot=[]  CS8Pos=[]  CS8Rot=[]  CS9Pos=[]  CS9Rot=[]  CS10Pos=[]  CS10Rot=[]  CS11Pos=[]  CS11Rot=[]  CS12Pos=[]  CS12Rot=[]  CS13Pos=[]  CS13Rot=[]  CS14Pos=[]  CS14Rot=[]  CS15Pos=[]  CS15Rot=[]  CS16Pos=[]  CS16Rot=[]  CS17Pos=[]  CS17Rot=[]  CS18Pos=[]  CS18Rot=[]  CS19Pos=[]  CS19Rot=[]  CS20Pos=[]  CS20Rot=[]
      settings: SourceProductName=Simscape Multibody  SourceProductBaseCode=MS
  "Torque " : Outport
  wires:
  Motion 1/1 -> Actuator2/1
  Motion 2/1 -> Actuator3/1
  Motion 3/1 -> Actuator4/1
  Motion 4/1 -> Actuator5/1
  Motion 5/1 -> Actuator6/1
  Joint 3 Sensor/1 -> Mux2/3
  Joint 6 Sensor/1 -> Mux2/6
  "Motion "/1 -> Actuator1/1
  Mux2/1 -> "Torque "/1
  Joint 1 Sensor/1 -> Mux2/1
  Joint 2 Sensor/1 -> Mux2/2
  Joint 4 Sensor/1 -> Mux2/4
  Joint 5 Sensor/1 -> Mux2/5
  connections:
  Actuator5/RConn1 -- Joint 5/LConn2
  Shoulder/RConn1 -- Joint 2/LConn1
  Joint 3 Sensor/LConn1 -- Joint 3/RConn2
  Weld/RConn1 -- Base/LConn1
  Joint 3/RConn1 -- Forarm/LConn1
  Joint 5/RConn1 -- Wrist-B/LConn1
  Joint 6/RConn1 -- Hand/LConn1
  Joint 6 Sensor/LConn1 -- Joint 6/RConn2
  Joint 2/RConn1 -- Arm/LConn1
  Actuator3/RConn1 -- Joint 3/LConn2
  Joint 5 Sensor/LConn1 -- Joint 5/RConn2
  Joint 4 Sensor/LConn1 -- Joint 4/RConn2
  Arm/RConn1 -- Joint 3/LConn1
  Actuator6/RConn1 -- Joint 6/LConn2
  Actuator4/RConn1 -- Joint 4/LConn2
  Joint 1/RConn1 -- Shoulder/LConn1
  RootPart/RConn1 -- Weld/LConn1
  Base/RConn1 -- Joint 1/LConn1
  Wrist-A/RConn1 -- Joint 5/LConn1
  Wrist-B/RConn1 -- Joint 6/LConn1
  Weld1/RConn1 -- RootPart/LConn1
  Joint 4/RConn1 -- Wrist-A/LConn1
  Forarm/RConn1 -- Joint 4/LConn1
  Joint 2 Sensor/LConn1 -- Joint 2/RConn2
  RootGround/RConn1 -- Weld1/LConn1
  Actuator2/RConn1 -- Joint 2/LConn2
  Joint 1/LConn2 -- Actuator1/RConn1
  Joint 1/RConn2 -- Joint 1 Sensor/LConn1
  Machine Environment/RConn1 -- RootGround/LConn1

== matlab function ImpedanceControl/MATLAB Function1 ==
  data: q input; We output; dq input
function We  = Jacobian_angular_velocities(q,dq)
%JACOBIANW
%    B = JACOBIANW(Q1,Q2,Q3,Q4,Q5)

%    This function was generated by the Symbolic Math Toolbox version 7.2.
%    23-Apr-2017 14:55:34

q=num2cell(q);
[q1,q2,q3,q4,q5,~]=deal(q{:});
%dq=num2cell(dq);
%[dq1,dq2,dq3,dq4,dq5,dq6]=deal(dq{:});

t2 = sin(q1);
t3 = cos(q1);
t4 = cos(q2);
t5 = sin(q3);
t6 = t3.*t4.*t5;
t7 = cos(q3);
t8 = sin(q2);
t13 = t3.*t7.*t8;
t9 = t6-t13;
t10 = pi.*(1.1e1./3.6e1);
t11 = sin(t10);
t12 = cos(t10);
t14 = t9.*t12;
t15 = cos(q4);
t16 = t2.*t11.*t15;
t17 = sin(q4);
t18 = t3.*t4.*t7;
t19 = t3.*t5.*t8;
t20 = t18+t19;
t21 = t11.*t17.*t20;
t22 = t14+t16+t21;
t23 = q2-q3;
t24 = sin(q5);
t25 = t2.*t17;
t26 = cos(q5);
t27 = t2.*t12.*t15;
t28 = sin(t23);
t29 = cos(t23);
t30 = t2.*t4.*t5;
t32 = t2.*t7.*t8;
t31 = t30-t32;
t33 = t12.*t31;
t34 = t2.*t5.*t8;
t35 = t2.*t4.*t7;
t36 = t34+t35;
t37 = t11.*t17.*t36;
t39 = t3.*t11.*t15;
t38 = t33+t37-t39;
t40 = t3.*t17;
t41 = t3.*t12.*t15;
t42 = t4.*t7;
t43 = t5.*t8;
t44 = t42+t43;
t45 = t12.*t44;
t46 = t4.*t5;
t49 = t7.*t8;
t47 = t46-t49;
t48 = t45-t11.*t17.*t47;
B = reshape([t2,-t3,0.0,-t2,t3,0.0,t9,t31,t44,t22,t38,t48,t12.*t22+t11.*t26.*(t27-t9.*t11+t12.*t17.*t20)-t11.*t24.*(t25-t15.*t20),t12.*t38-t11.*t26.*(t41+t11.*t31-t12.*t17.*t36)+t11.*t24.*(t40+t15.*t36),t12.*t48-t11.*t26.*(t11.*t44+t12.*t17.*t47)-t11.*t15.*t24.*t47,-t12.*(t16-t3.*t12.*t28+t3.*t11.*t17.*t29)-t11.*t26.*(t27+t3.*t11.*t28+t3.*t12.*t17.*t29)-t11.*t24.*(-t25+t3.*t4.*t7.*t15+t3.*t5.*t8.*t15),t12.*(t39+t2.*t12.*t28-t2.*t11.*t17.*t29)-t11.*t26.*(-t41+t2.*t11.*t28+t2.*t12.*t17.*t29)-t11.*t24.*(t40+t2.*t4.*t7.*t15+t2.*t5.*t8.*t15),-t12.*(t12.*t29+t11.*t17.*t28)+t11.*t26.*(t11.*t29-t12.*t17.*t28)-t11.*t15.*t24.*t28],[3,6]);
We=B*dq;

== matlab function ImpedanceControl/MATLAB Function ==
  data: q input; Oe output; Re output
function [ Oe, Re ] = DirectKinematics(q)
% DirectKinematics
%    [ Oe, Re ] = DirectKinematics(q)
%    This function was generated by the Symbolic Math Toolbox version 7.2.
%    23-Apr-2017 13:45:31

q=num2cell(q);
[q1,q2,q3,q4,q5,q6]=deal(q{:});

t2 = q1+q2;
t3 = cos(t2);
t4 = q3+q4;
t5 = sin(t2);
t6 = cos(q5);
t7 = cos(t4);
t8 = sin(q5);
t9 = sin(q6);
t10 = cos(q6);
t11 = sin(t4);
t12 = t3.*t11.*4.698463103929542e-1;
t13 = t3.*t7.*t8.*4.698463103929542e-1;
t14 = t5.*t11.*4.698463103929542e-1;
t15 = t3.*t8;
t16 = t15-t5.*t6.*t7;
t17 = t3.*t6.*4.698463103929542e-1;
t18 = t5.*t7.*t8.*4.698463103929542e-1;
t19 = cos(q3);
T06 = reshape([t10.*(t5.*t8+t3.*t6.*t7)-t9.*(t5.*t6.*(-5.735764363510462e-1)+t3.*t11.*8.191520442889917e-1+t3.*t7.*t8.*5.735764363510462e-1),-t10.*t16-t9.*(t3.*t6.*5.735764363510462e-1+t5.*t11.*8.191520442889917e-1+t5.*t7.*t8.*5.735764363510462e-1),t7.*t9.*(-8.191520442889917e-1)-t6.*t10.*t11+t8.*t9.*t11.*5.735764363510462e-1,0.0,-t12-t10.*(t12-t5.*t6.*3.289899283371657e-1+t3.*t7.*t8.*3.289899283371657e-1)-t9.*(t5.*t8.*5.735764363510462e-1+t3.*t6.*t7.*5.735764363510462e-1)-t5.*t6.*6.710100716628342e-1+t3.*t7.*t8.*6.710100716628342e-1,-t14-t10.*(t14+t3.*t6.*3.289899283371657e-1+t5.*t7.*t8.*3.289899283371657e-1)+t9.*(t3.*t8.*5.735764363510462e-1-t5.*t6.*t7.*5.735764363510462e-1)+t3.*t6.*6.710100716628342e-1+t5.*t7.*t8.*6.710100716628342e-1,t7.*(-4.698463103929542e-1)-t7.*t10.*4.698463103929542e-1-t8.*t11.*6.710100716628342e-1+t6.*t9.*t11.*5.735764363510462e-1+t8.*t10.*t11.*3.289899283371657e-1,0.0,t13+t10.*(t13-t5.*t6.*4.698463103929542e-1+t3.*t11.*6.710100716628342e-1)-t5.*t6.*4.698463103929542e-1-t3.*t11.*3.289899283371657e-1+t9.*(t5.*t8.*8.191520442889917e-1+t3.*t6.*t7.*8.191520442889917e-1),t17+t18-t5.*t11.*3.289899283371657e-1-t9.*t16.*8.191520442889917e-1+t10.*(t17+t18+t5.*t11.*6.710100716628342e-1),t7.*(-3.289899283371657e-1)+t7.*t10.*6.710100716628342e-1-t8.*t11.*4.698463103929542e-1-t6.*t9.*t11.*8.191520442889917e-1-t8.*t10.*t11.*4.698463103929542e-1,0.0,t5.*(-2.589822393260846e-1)-t5.*t6.*1.724988718349159e-1-t3.*t11.*2.04549489043648e-1+t3.*t19.*(4.1e1./1.0e2)+t3.*t7.*t8.*1.724988718349159e-1,t3.*2.589822393260846e-1+t3.*t6.*1.724988718349159e-1-t5.*t11.*2.04549489043648e-1+t5.*t19.*(4.1e1./1.0e2)+t5.*t7.*t8.*1.724988718349159e-1,t7.*(-2.04549489043648e-1)-sin(q3).*(4.1e1./1.0e2)-t8.*t11.*1.724988718349159e-1+2.755e-1,1.0],[4,4]);
Re=T06(1:3,1:3);
Oe=T06(1:3,4);

== matlab function ImpedanceControl/MATLAB Function2 ==
  data: q input; dOe output; dq input
function dOe = PositionDerivative(q,dq)
%POSITIONDERIVATIVE
%    DOE = POSITIONDERIVATIVE(DQ1,DQ2,DQ3,DQ4,DQ5,Q1,Q2,Q3,Q4,Q5)

%    This function was generated by the Symbolic Math Toolbox version 7.2.
%    23-Apr-2017 15:43:12

q=num2cell(q);
dq=num2cell(dq);
[q1,q2,q3,q4,q5,q6]=deal(q{:});
[dq1,dq2,dq3,dq4,dq5,dq6]=deal(dq{:});

t2 = q1+q2;
t3 = dq1+dq2;
t4 = cos(t2);
t5 = pi.*(1.1e1./7.2e1);
t6 = cos(t5);
t7 = sin(t2);
t8 = pi.*(1.1e1./3.6e1);
t9 = sin(t8);
t10 = cos(t8);
t11 = q3+q4;
t12 = cos(t11);
t13 = cos(q5);
t14 = sin(q5);
t15 = sin(t11);
t16 = dq3+dq4;
t17 = 1.0./t6;
t18 = cos(q3);
t19 = sin(q3);
t20 = t6.*3.374e3;
t21 = t20+7.43e2;
t22 = t6.*4.146e3;
t23 = t22+7.43e2;
t24 = sin(t5);
dOe = [t3.*t4.*(-9.8e-3)-t17.*t21.*(-dq5.*t7.*t9.*t14+t3.*t4.*t9.*t13-t3.*t7.*t10.*t15+t4.*t10.*t12.*t16-dq5.*t4.*t9.*t12.*t13+t3.*t7.*t9.*t12.*t14+t4.*t9.*t14.*t15.*t16).*5.0e-5-dq3.*t4.*t19.*(4.1e1./1.0e2)-t3.*t7.*t18.*(4.1e1./1.0e2)+t3.*t7.*t15.*t17.*7.43e-2-t3.*t4.*t17.*t23.*5.0e-5-t4.*t12.*t16.*t17.*7.43e-2;t3.*t7.*(-9.8e-3)-t17.*t21.*(dq5.*t4.*t9.*t14+t3.*t4.*t10.*t15+t3.*t7.*t9.*t13+t7.*t10.*t12.*t16-dq5.*t7.*t9.*t12.*t13-t3.*t4.*t9.*t12.*t14+t7.*t9.*t14.*t15.*t16).*5.0e-5-dq3.*t7.*t19.*(4.1e1./1.0e2)+t3.*t4.*t18.*(4.1e1./1.0e2)-t3.*t4.*t15.*t17.*7.43e-2-t3.*t7.*t17.*t23.*5.0e-5-t7.*t12.*t16.*t17.*7.43e-2;dq3.*t18.*(-4.1e1./1.0e2)-t17.*t21.*(-t15.*t16.*(t6.^2.*2.0-1.0)+dq5.*t6.*t13.*t15.*t24.*2.0+t6.*t12.*t14.*t16.*t24.*2.0).*5.0e-5+t15.*t16.*t17.*7.43e-2];
